simulink model "VehicleDynamics3D_traj"  (R2018a)
settings: Solver=ode15s  StartTime=0.0  StopTime=Stoptime  FixedStep=.001  MaxStep=maxStep  RelTol=relTol  AbsTol=absTol  EnableMultiTasking=on
PreLoadFcn:
  | VehicleDynamicsInitialization.m
model workspace: external: MATLAB File C:\Users\Puspita\Desktop\VehicleDynamics\sm_suspension_templates_params_ori.m (data not in the file)
values from neighbouring files (symbols this model uses):
  contactDamping = 1200    [VehicleDynamicsInitialization.m]    (also in traj1_results.mat)
  contactStiffness = 1E+6    (= 1000000)    [VehicleDynamicsInitialization.m]    (also in traj1_results.mat)
  dwb =     [modelworkspace.mat]    (also in sm_suspension_templates_params_ref.m = struct)
  Floor =     [traj1_results.mat]
  followerCameraX = 7.5    [VehicleDynamicsInitialization.m]    (also in traj1_results.mat)
  followerCameraZ = 3    [VehicleDynamicsInitialization.m]    (also in traj1_results.mat)
  frontCameraX = -1.75    [VehicleDynamicsInitialization.m]    (also in traj1_results.mat)
  frontCameraZ = 0.35    [VehicleDynamicsInitialization.m]    (also in traj1_results.mat)
  isoCameraAimX = (1/2)*wheelbase    (= 0.75)    [VehicleDynamicsInitialization.m]    (also in traj1_results.mat)
  isoCameraX = -3.1    [VehicleDynamicsInitialization.m]    (also in traj1_results.mat)
  isoCameraY = 3.5    [VehicleDynamicsInitialization.m]    (also in traj1_results.mat)
  isoCameraZ = 1.5    [VehicleDynamicsInitialization.m]    (also in traj1_results.mat)
  kineticFrictionCoeff = 0.88    [VehicleDynamicsInitialization.m]    (also in traj1_results.mat)
  limit = 105    [Run_Rear_Ident.m]    (also in test_traj.m = 50; traj1_results.mat = 50)
  Load = 200*scale    (= 200)    [VehicleDynamicsInitialization.m]    (also in traj1_results.mat)
  m = 200    [test_2.mat]    (also in test_traj.mat; test_traj2.mat; traj1_results.mat; traj_8.mat)
  maxSteeringDisplacement = 12    [VehicleDynamicsInitialization.m]    (also in traj1_results.mat = 10)
  minSteeringDisplacement = -12    [VehicleDynamicsInitialization.m]    (also in traj1_results.mat = -10)
  SetPaceSampleTime = 0.1    [VehicleDynamicsInitialization.m]    (also in traj1_results.mat)
  staticFrictionCoeff = 0.90    (= 0.9)    [VehicleDynamicsInitialization.m]    (also in traj1_results.mat)
  steeringInput = 0    [VehicleDynamicsInitialization.m]    (also in traj1_results.mat)
  vehicleSpeed_kph = 0    [VehicleDynamicsInitialization.m]    (also in traj1_results.mat)
  velocityThreshold = 1.5    [VehicleDynamicsInitialization.m]    (also in traj1_results.mat)
  wheel =     [modelworkspace.mat]    (also in sm_suspension_templates_params_ref.m = struct; traj1_results.mat)
  wheelbase = 1.5*scale    (= 1.5)    [VehicleDynamicsInitialization.m]    (also in traj1_results.mat)
undefined symbols (not defined in the file or in its folder): sigbuilder_block, X, Y, Z
libraries: sm_lib x237, nesl_utility x83, sm_suspension_templates_lib x34, Contact_Forces_Lib x16, simulink x12, fl_lib x1, aerolibanimutils x1
(part 5 of 10)

== system VehicleDynamics3D_traj/FrontSuspension/Chassis Assembly ==
  Back Frame : sm_suspension_templates_lib/Trapezoidal Frame  L1=dwb.chassis.frame.longlength  L2=dwb.chassis.frame.shortlength  H=dwb.chassis.frame.height  R=dwb.chassis.frame.cornerradius  T=dwb.chassis.frame.thickness  Tb=dwb.chassis.frame.barthickness  rho=dwb.chassis.frame.density  clr=dwb.chassis.frame.color
  DL Link : sm_suspension_templates_lib/Link 3  L=dwb.chassis.lowerlink.length  Ro=dwb.chassis.lowerlink.outerradius  Ri=dwb.chassis.lowerlink.innerradius  Lw=dwb.chassis.lowerlink.wishboneslotlength  Ld=dwb.chassis.lowerlink.wishboneseparation  Ow=dwb.chassis.lowerlink.wishboneoffset  Rr=dwb.chassis.lowerlink.chamferradius  rho=dwb.chassis.lowerlink.density  clr=dwb.chassis.lowerlink.color
  DR Link : sm_suspension_templates_lib/Link 3  L=dwb.chassis.lowerlink.length  Ro=dwb.chassis.lowerlink.outerradius  Ri=dwb.chassis.lowerlink.innerradius  Lw=dwb.chassis.lowerlink.wishboneslotlength  Ld=dwb.chassis.lowerlink.wishboneseparation  Ow=dwb.chassis.lowerlink.wishboneoffset  Rr=dwb.chassis.lowerlink.chamferradius  rho=dwb.chassis.lowerlink.density  clr=dwb.chassis.lowerlink.color
  Front Frame : Subsystem  mask(Trapeziodal Frame){L1=dwb.chassis.frame.longlength, L2=dwb.chassis.frame.shortlength, H=dwb.chassis.frame.height, R=dwb.chassis.frame.cornerradius, T=dwb.chassis.frame.thickness, Tb=dwb.chassis.frame.barthickness, rho=dwb.chassis.frame.density, clr=dwb.chassis.frame.color}
      mask prompts: L1 "Long side length of frame (cm):"; L2 "Short side length of frame (cm):"; H "Height of frame (cm):"; R "Radius of rounded corners (cm):"; T "Thickness of frame (cm):"; Tb "Thickness of frame bars (cm):"; rho "Density (kg/m^3):"; clr "Color ([r g b]):"
      mask help: This block models a trapeziodal frame that is part of the chassis on to which the suspension is mounted. The ports DR, DL, UR, UL correspond to the four corners of the frame. The port R corresponds to the central reference frame.
      mask init:
      | phi = atan2(H,(L1-L2)/2);
      | 
      | outer_xsec = [L2/2 -H/2; L1/2 H/2; -L1/2 H/2; -L2/2 -H/2];
      | 
      | inner_xsec = [ L2/2-Tb/tan((pi-phi)/2)    -(H/2-Tb);
      |                -L2/2+Tb/tan((pi-phi)/2)   -(H/2-Tb);
      |                -L1/2+Tb/tan(phi/2)          H/2-Tb;
      |                L1/2-Tb/tan(phi/2)           H/2-Tb];
      | 
      | % Frames are midway between the inner and outer 
      | % trapezium vertices           
      | frames = (outer_xsec+[inner_xsec(1,:); flipud(inner_xsec(2:end,:))])/2;
      | 
      | outer_xsec = simmechanics.demohelpers.round_corners(outer_xsec,[1 2 3 4],R,20);
      | inner_xsec = simmechanics.demohelpers.round_corners(inner_xsec,[1 2 3 4],R,20);       
      |           
      | frame_xsec = [outer_xsec; outer_xsec(1,:); ...
      |               inner_xsec; inner_xsec(1,:)];      
      |           
      | sec = frames(1,:);          
      | nec = frames(2,:);          
      | nwc = frames(3,:);          
      | swc = frames(4,:);
      mask DialogControl ParameterTabVar0 Prompt: Dimensions
      mask DialogControl ParameterTabVar01 Prompt: Material Properties
      mask Display:
      | image(imread(fullfile(matlabroot,...
      |     'toolbox','physmod','sm','smdemos',...
      |     'suspension_templates','images','sm_isuspension_frame.png')));
      | 
      | port_label('LConn',1,'UL');
      | port_label('LConn',2,'DL');
      | port_label('LConn',3,'DR');
      | port_label('LConn',4,'UR');
  Load : Subsystem
  NE Damp Joint : sm_lib/Joints/Revolute Joint  SenseConstraintForce=off  SenseConstraintForceX=off  SenseConstraintForceY=off  SenseConstraintForceZ=off  SenseConstraintTorque=off  SenseConstraintTorqueX=off  SenseConstraintTorqueY=off  SenseConstraintTorqueZ=off  SenseTotalForce=off  SenseTotalForceX=off  SenseTotalForceY=off  SenseTotalForceZ=off  SenseTotalTorque=off  SenseTotalTorqueX=off  SenseTotalTorqueY=off  SenseTotalTorqueZ=off  CompositeWrenchDir=FollowerOnBase  CompositeWrenchFrame=BaseFrame  EquilibriumPosition=0  EquilibriumPositionUnits=deg  SpringStiffness=0  SpringStiffnessUnits=N*m/deg  DampingCoefficient=0  DampingCoefficientUnits=N*m/(deg/s)  TorqueActuationMode=NoTorque  MotionActuationMode=ComputedMotion  SensePosition=off  SenseVelocity=off  SenseAcceleration=off  SenseTorqueForce=off  PositionTargetSpecify=off  PositionTargetPriority=High  PositionTargetValue=0  PositionTargetValueUnits=deg  VelocityTargetSpecify=off  VelocityTargetPriority=High  VelocityTargetValue=0  VelocityTargetValueUnits=deg/s
  NW Damp Joint : sm_lib/Joints/Revolute Joint  SenseConstraintForce=off  SenseConstraintForceX=off  SenseConstraintForceY=off  SenseConstraintForceZ=off  SenseConstraintTorque=off  SenseConstraintTorqueX=off  SenseConstraintTorqueY=off  SenseConstraintTorqueZ=off  SenseTotalForce=off  SenseTotalForceX=off  SenseTotalForceY=off  SenseTotalForceZ=off  SenseTotalTorque=off  SenseTotalTorqueX=off  SenseTotalTorqueY=off  SenseTotalTorqueZ=off  CompositeWrenchDir=FollowerOnBase  CompositeWrenchFrame=BaseFrame  EquilibriumPosition=0  EquilibriumPositionUnits=deg  SpringStiffness=0  SpringStiffnessUnits=N*m/deg  DampingCoefficient=0  DampingCoefficientUnits=N*m/(deg/s)  TorqueActuationMode=NoTorque  MotionActuationMode=ComputedMotion  SensePosition=off  SenseVelocity=off  SenseAcceleration=off  SenseTorqueForce=off  PositionTargetSpecify=off  PositionTargetPriority=High  PositionTargetValue=0  PositionTargetValueUnits=deg  VelocityTargetSpecify=off  VelocityTargetPriority=High  VelocityTargetValue=0  VelocityTargetValueUnits=deg/s
  Steering System : Subsystem
      mask Display:
      | image(imread(fullfile(matlabroot,...
      |     'toolbox','physmod','sm','smdemos',...
      |     'suspension_templates','images','sm_isuspension_steeringsys.png')))
      | 
      | port_label('LConn',1,'B');
      | port_label('RConn',1,'LT');
      | port_label('RConn',2,'RT');
  UL Link : sm_suspension_templates_lib/Link 1  L=dwb.chassis.upperlink.length  Ro=dwb.chassis.upperlink.outerradius  Ri=dwb.chassis.upperlink.innerradius  Lw=dwb.chassis.upperlink.wishboneslotlength  Ls=dwb.chassis.upperlink.springdamperslotlength  Ld=dwb.chassis.upperlink.wishboneseparation  Ow=dwb.chassis.upperlink.wishboneoffset  Rr=dwb.chassis.upperlink.chamferradius  rho=dwb.chassis.upperlink.density  clr=dwb.chassis.upperlink.color
  UR Link : sm_suspension_templates_lib/Link 1  L=dwb.chassis.upperlink.length  Ro=dwb.chassis.upperlink.outerradius  Ri=dwb.chassis.upperlink.innerradius  Lw=dwb.chassis.upperlink.wishboneslotlength  Ls=dwb.chassis.upperlink.springdamperslotlength  Ld=dwb.chassis.upperlink.wishboneseparation  Ow=dwb.chassis.upperlink.wishboneoffset  Rr=dwb.chassis.upperlink.chamferradius  rho=dwb.chassis.upperlink.density  clr=dwb.chassis.upperlink.color
  BC : PMIOPort  Side=Left
  ULA : PMIOPort  Port=2  Side=Left
  ULB : PMIOPort  Port=3  Side=Left
  ULC : PMIOPort  Port=4  Side=Left
  DLA : PMIOPort  Port=5  Side=Left
  DLB : PMIOPort  Port=6  Side=Left
  LT : PMIOPort  Port=7  Side=Left
  URA : PMIOPort  Port=8  Side=Right
  URB : PMIOPort  Port=9  Side=Right
  URC : PMIOPort  Port=10  Side=Right
  DRA : PMIOPort  Port=11  Side=Right
  DRB : PMIOPort  Port=12  Side=Right
  RT : PMIOPort  Port=13  Side=Right
  S : PMIOPort  Port=14  Side=Left
  connections:
  DR Link/LConn3 -- DRB/RConn1
  DR Link/LConn2 -- DRA/RConn1
  DLA/RConn1 -- DL Link/LConn2
  DLB/RConn1 -- DL Link/LConn3
  UR Link/LConn3 -- URB/RConn1
  UR Link/LConn2 -- URA/RConn1
  Front Frame/LConn2 -- DL Link/LConn1
  UR Link/LConn1 -- Front Frame/LConn4
  Back Frame/LConn2 -- DL Link/LConn4
  DR Link/LConn1 -- Front Frame/LConn3
  ULB/RConn1 -- UL Link/LConn3
  Back Frame/LConn3 -- DR Link/LConn4
  UR Link/LConn5 -- Back Frame/LConn4
  Back Frame/LConn1 -- UL Link/LConn5
  ULA/RConn1 -- UL Link/LConn2
  UL Link/LConn1 -- Front Frame/LConn1
  Back Frame/RConn1 -- Load/RConn1 -- Steering System/LConn1 -- BC/RConn1
  LT/RConn1 -- Steering System/RConn1
  Steering System/RConn2 -- RT/RConn1
  NW Damp Joint/LConn1 -- UL Link/LConn4
  NW Damp Joint/RConn1 -- ULC/RConn1
  NE Damp Joint/LConn1 -- UR Link/LConn4
  NE Damp Joint/RConn1 -- URC/RConn1
  S/RConn1 -- Steering System/LConn2

== system VehicleDynamics3D_traj/FrontSuspension/L Spr-Damp Assm ==
  Cyl Bracket : sm_suspension_templates_lib/Single Bracket  L=Lb  W=Wb  T=Tb  Rh=Rbh  rho=rho  clr=cclr
  Cyl Bracket XForm : sm_lib/Frames and Transforms/Rigid Transform  TranslationMethod=StandardAxis  TranslationStandardOffset=Lc/2  TranslationLengthUnit=cm  TranslationStandardAxis=-Z  TranslationCartesianOffset=[0 0 0]  TranslationROffset=0  TranslationROffsetUnits=m  TranslationZOffset=0  TranslationZOffsetUnits=m  TranslationThetaOffset=0  TranslationThetaOffsetUnits=deg  RotationMethod=AlignedAxes  RotationAngleUnits=deg  RotationStandardAxis=+Z  RotationAngle=0  RotationArbitraryAxis=[0 0 1]  FollAlignAxisA=+Z  BaseAlignAxisA=-Z  FollAlignAxisB=+X  BaseAlignAxisB=-X  RotationSequenceAxes=FollowerAxes  RotationSequence=XYX  RotationSequenceAngles=[0 0 0]  RotationSequenceAnglesUnits=deg  RotationMatrix=[1 0 0; 0 1 0; 0 0 1]
  Cyl-Piston Joint : sm_lib/Joints/Prismatic Joint  SenseConstraintForce=off  SenseConstraintForceX=off  SenseConstraintForceY=off  SenseConstraintForceZ=off  SenseConstraintTorque=off  SenseConstraintTorqueX=off  SenseConstraintTorqueY=off  SenseConstraintTorqueZ=off  SenseTotalForce=off  SenseTotalForceX=off  SenseTotalForceY=off  SenseTotalForceZ=off  SenseTotalTorque=off  SenseTotalTorqueX=off  SenseTotalTorqueY=off  SenseTotalTorqueZ=off  CompositeWrenchDir=FollowerOnBase  CompositeWrenchFrame=BaseFrame  EquilibriumPosition=Ls-(Lc-Lp)/2  EquilibriumPositionUnits=cm  SpringStiffness=Ks  SpringStiffnessUnits=N/m  DampingCoefficient=Kb  DampingCoefficientUnits=N/(m/s)  TorqueActuationMode=NoTorque  MotionActuationMode=ComputedMotion  SensePosition=on  SenseVelocity=off  SenseAcceleration=off  SenseTorqueForce=off  PositionTargetSpecify=off  PositionTargetPriority=Low  PositionTargetValue=Lp/2  PositionTargetValueUnits=cm  VelocityTargetSpecify=off  VelocityTargetPriority=High  VelocityTargetValue=0  VelocityTargetValueUnits=m/s
  Cylinder : sm_lib/Body Elements/Solid  InertiaType=CalculateFromGeometry  Mass=1  MassUnits=kg  CenterOfMass=[0 0 0]  CenterOfMassUnits=m  MomentsOfInertia=[1 1 1]  MomentsOfInertiaUnits=kg*m^2  ProductsOfInertia=[0 0 0]  ProductsOfInertiaUnits=kg*m^2  DensityBased=on  Density=rho  DensityUnits=kg/(m^3)  DoExposeReferenceFrame=on  SerializedFrames=<Frames/>  GraphicType=FromGeometry  MarkerShape=Sphere  MarkerSize=10  MarkerSizeUnits=m  GraphicVisPropType=SimpleVisualProperties  GraphicDiffuseColor=cclr  GraphicSpecularColor=[0.5 0.5 0.5 1.0]  GraphicAmbientColor=[0.15 0.15 0.15 1.0]  GraphicEmissiveColor=[0.0 0.0 0.0 1.0]  GraphicShininess=75  GraphicOpacity=0.75  GeometryShape=GeneralSolidOfRevolution  RectangleSize=[1 1]  RectangleSizeUnits=m  BrickDimensions=[1 1 1]  BrickDimensionUnits=m  CylinderRadius=1  CylinderRadiusUnits=m  CylinderLength=1  CylinderLengthUnits=m  SphereRadius=1  SphereRadiusUnits=m  EllipsoidRadii=[1 1 1]  EllipsoidRadiiUnits=m  ExtrusionCrossSection=[1 1; -1 1; -1 -1; 1 -1]  ExtrusionCrossSectionUnits=m  ExtrusionLength=1  ExtrusionLengthUnits=m  PolygonNumSides=3  PolygonOuterRadius=1  PolygonOuterRadiusUnits=m  ExtGeomFileType=STL  ExtGeomFileUnits=m  RevolutionCrossSection=cyl_xsec  RevolutionCrossSectionUnits=cm  RevolutionExtent=Full  RevolutionAngle=180  RevolutionAngleUnits=deg
  PS-Simulink Converter : nesl_utility/PS-Simulink Converter  PhysicalDomain=network_engine_domain  SubClassName=ps_output  LeftPortType=input  RightPortType=output  PseudoPeriodic=off  Frequencies=[]  Unit=cm  AffineConversion=off
  Pistion Bracket : sm_suspension_templates_lib/Single Bracket  L=Lb  W=Wb  T=Tb  Rh=Rbh  rho=rho  clr=pclr
  Piston : sm_lib/Body Elements/Solid  InertiaType=CalculateFromGeometry  Mass=1  MassUnits=kg  CenterOfMass=[0 0 0]  CenterOfMassUnits=m  MomentsOfInertia=[1 1 1]  MomentsOfInertiaUnits=kg*m^2  ProductsOfInertia=[0 0 0]  ProductsOfInertiaUnits=kg*m^2  DensityBased=on  Density=rho  DensityUnits=kg/(m^3)  DoExposeReferenceFrame=on  SerializedFrames=<Frames/>  GraphicType=FromGeometry  MarkerShape=Sphere  MarkerSize=10  MarkerSizeUnits=m  GraphicVisPropType=SimpleVisualProperties  GraphicDiffuseColor=pclr  GraphicSpecularColor=[0.5 0.5 0.5 1.0]  GraphicAmbientColor=[0.15 0.15 0.15 1.0]  GraphicEmissiveColor=[0.0 0.0 0.0 1.0]  GraphicShininess=75  GraphicOpacity=1  GeometryShape=GeneralSolidOfRevolution  RectangleSize=[1 1]  RectangleSizeUnits=m  BrickDimensions=[1 1 1]  BrickDimensionUnits=m  CylinderRadius=1  CylinderRadiusUnits=m  CylinderLength=1  CylinderLengthUnits=m  SphereRadius=1  SphereRadiusUnits=m  EllipsoidRadii=[1 1 1]  EllipsoidRadiiUnits=m  ExtrusionCrossSection=[1 1; -1 1; -1 -1; 1 -1]  ExtrusionCrossSectionUnits=m  ExtrusionLength=1  ExtrusionLengthUnits=m  PolygonNumSides=3  PolygonOuterRadius=1  PolygonOuterRadiusUnits=m  ExtGeomFileType=STL  ExtGeomFileUnits=m  RevolutionCrossSection=piston_xsec  RevolutionCrossSectionUnits=cm  RevolutionExtent=Full  RevolutionAngle=180  RevolutionAngleUnits=deg
  Piston Bracket XForm : sm_lib/Frames and Transforms/Rigid Transform  TranslationMethod=StandardAxis  TranslationStandardOffset=Lp/2  TranslationLengthUnit=cm  TranslationStandardAxis=+Z  TranslationCartesianOffset=[0 0 0]  TranslationROffset=0  TranslationROffsetUnits=m  TranslationZOffset=0  TranslationZOffsetUnits=m  TranslationThetaOffset=0  TranslationThetaOffsetUnits=deg  RotationMethod=None  RotationAngleUnits=deg  RotationStandardAxis=+Z  RotationAngle=0  RotationArbitraryAxis=[0 0 1]  FollAlignAxisA=+Z  BaseAlignAxisA=+Z  FollAlignAxisB=+X  BaseAlignAxisB=-X  RotationSequenceAxes=FollowerAxes  RotationSequence=XYX  RotationSequenceAngles=[0 0 0]  RotationSequenceAnglesUnits=deg  RotationMatrix=[1 0 0; 0 1 0; 0 0 1]
  Terminator : Terminator
  P : PMIOPort  Side=Right
  C : PMIOPort  Port=2  Side=Left
  wires:
  PS-Simulink Converter/1 -> Terminator/1  "FLSuspensionTravel_cm"
  connections:
  C/RConn1 -- Cyl Bracket/LConn1
  Pistion Bracket/LConn1 -- P/RConn1
  Pistion Bracket/RConn1 -- Piston Bracket XForm/RConn1
  Cyl Bracket/RConn1 -- Cyl Bracket XForm/RConn1
  Cyl-Piston Joint/RConn1 -- Piston/RConn1 -- Piston Bracket XForm/LConn1
  Cylinder/RConn1 -- Cyl-Piston Joint/LConn1 -- Cyl Bracket XForm/LConn1
  Cyl-Piston Joint/RConn2 -- PS-Simulink Converter/LConn1

== system VehicleDynamics3D_traj/FrontSuspension/L Suspension Assembly ==
  Knuckle : sm_suspension_templates_lib/Knuckle  H=dwb.knuckle.height  L=dwb.knuckle.length  T=dwb.knuckle.thickness  Wpr=dwb.knuckle.wheelattachprojwidth  Hpr=dwb.knuckle.wheelattachprojheight  Wc=dwb.knuckle.wishboneconnectorwidth  Rd=dwb.knuckle.driveshaftradius  Hd=dwb.knuckle.driveshaftheight  Rr=dwb.knuckle.chamferradius  Rt=dwb.knuckle.transitionradius  Rb=dwb.knuckle.ball.radius  Rp=dwb.knuckle.pin.radius  Hp=dwb.knuckle.pin.height  Ls=dwb.knuckle.steerarm.length  Ws=dwb.knuckle.steerarm.width  Ts=dwb.knuckle.steerarm.thickness  Hsf=dwb.knuckle.steerarm.forkheight  Lsf=dwb.knuckle.steerarm.forklength  Osf=dwb.knuckle.steerarm.forkoffset  Rsp=dwb.knuckle.pinradius  Rsr=dwb.knuckle.chamferradius  Rev=on  rho=dwb.knuckle.density  clr=dwb.knuckle.color
  Lower Knuckle Joint : sm_lib/Joints/Spherical Joint  SenseConstraintForce=off  SenseConstraintForceX=off  SenseConstraintForceY=off  SenseConstraintForceZ=off  SenseConstraintTorque=off  SenseConstraintTorqueX=off  SenseConstraintTorqueY=off  SenseConstraintTorqueZ=off  SenseTotalForce=off  SenseTotalForceX=off  SenseTotalForceY=off  SenseTotalForceZ=off  SenseTotalTorque=off  SenseTotalTorqueX=off  SenseTotalTorqueY=off  SenseTotalTorqueZ=off  CompositeWrenchDir=FollowerOnBase  CompositeWrenchFrame=BaseFrame  DefPosRotationMethod=None  DefPosRotationAngleUnits=deg  DefPosRotationStandardAxis=+Z  DefPosRotationAngle=0  DefPosRotationArbitraryAxis=[0 0 1]  DefPosFollAlignAxisA=+X  DefPosBaseAlignAxisA=+Y  DefPosFollAlignAxisB=+Y  DefPosBaseAlignAxisB=+Z  DefPosRotationSequenceAxes=FollowerAxes  DefPosRotationSequence=XYX  DefPosRotationSequenceAngles=[0 0 0]  DefPosRotationSequenceAnglesUnits=deg  DefPosRotationMatrix=[1 0 0; 0 1 0; 0 0 1]  EqPosRotationMethod=None  EqPosRotationAngleUnits=deg  EqPosRotationStandardAxis=+Z  EqPosRotationAngle=0  EqPosRotationArbitraryAxis=[0 0 1]  EqPosFollAlignAxisA=+X  EqPosBaseAlignAxisA=+Y  EqPosFollAlignAxisB=+Y  EqPosBaseAlignAxisB=+Z  EqPosRotationSequenceAxes=FollowerAxes  EqPosRotationSequence=XYX  EqPosRotationSequenceAngles=[0 0 0]  EqPosRotationSequenceAnglesUnits=deg  EqPosRotationMatrix=[1 0 0; 0 1 0; 0 0 1]  SpringStiffness=0  SpringStiffnessUnits=N*m/deg  DampingCoefficient=0  DampingCoefficientUnits=N*m/(deg/s)  ActuateTorqueX=off  ActuateTorqueY=off  ActuateTorqueZ=off  ActuateTorque=off  TorqueActuationMode=NoTorque  MotionActuationMode=ComputedMotion  ActuationFrame=BaseFrame  SensePosition=off  SenseVelocityX=off  SenseVelocityY=off  SenseVelocityZ=off  SenseVelocity=off  SenseAccelerationX=off  SenseAccelerationY=off  SenseAccelerationZ=off  SenseAcceleration=off  SenseTorqueX=off  SenseTorqueY=off  SenseTorqueZ=off  SenseTorqueForce=off  SensingFrame=BaseFrame  PositionTargetRotationMethod=None  PositionTargetRotationAngleUnits=deg  PositionTargetRotationStandardAxis=+Z  PositionTargetRotationAngle=0  PositionTargetRotationArbitraryAxis=[0 0 1]  PositionTargetFollAlignAxisA=+Y  PositionTargetBaseAlignAxisA=-Y  PositionTargetFollAlignAxisB=+Z  PositionTargetBaseAlignAxisB=-Z  PositionTargetRotationSequenceAxes=FollowerAxes  PositionTargetRotationSequence=XYX  PositionTargetRotationSequenceAngles=[0 0 0]  PositionTargetRotationSequenceAnglesUnits=deg  PositionTargetRotationMatrix=[1 0 0; 0 1 0; 0 0 1]  PositionTargetSpecify=off  PositionTargetPriority=Low  VelocityTargetValue=[0 0 0]  VelocityTargetValueUnits=deg/s  VelocityTargetSpecify=off  VelocityTargetPriority=High  VelocityTargetInFollowerFrame=on
  Lower Wishbone : sm_suspension_templates_lib/Lower Wishbone  L1=dwb.lwb.longlength  L2=dwb.lwb.shortlength  L3=dwb.lwb.wheellinklength  W3=dwb.lwb.wheellinkwidth  W=dwb.lwb.width  T=dwb.lwb.thickness  Rb=dwb.lwb.baseradius  Ob=dwb.lwb.basearcoffset  Rev=on  Lb=dwb.lwb.bracket.length  Rsh=dwb.lwb.bracket.radius  Rs=dwb.lwb.socket.radius  Hi=dwb.lwb.socket.height  Rh=dwb.lwb.socket.holeradius  Oh=dwb.lwb.socket.holeoffset  Odb=dwb.lwb.damperbracket.offset  Wdb=dwb.lwb.damperbracket.width  Ldb=dwb.lwb.damperbracket.length  Tdb=dwb.lwb.damperbracket.thickness  Sdb=dwb.lwb.damperbracket.spacing  Rhdb=dwb.lwb.damperbracket.holeradius  rho=dwb.lwb.density  clr=dwb.lwb.color
  SW Damp Joint : sm_lib/Joints/Revolute Joint  SenseConstraintForce=off  SenseConstraintForceX=off  SenseConstraintForceY=off  SenseConstraintForceZ=off  SenseConstraintTorque=off  SenseConstraintTorqueX=off  SenseConstraintTorqueY=off  SenseConstraintTorqueZ=off  SenseTotalForce=off  SenseTotalForceX=off  SenseTotalForceY=off  SenseTotalForceZ=off  SenseTotalTorque=off  SenseTotalTorqueX=off  SenseTotalTorqueY=off  SenseTotalTorqueZ=off  CompositeWrenchDir=FollowerOnBase  CompositeWrenchFrame=BaseFrame  EquilibriumPosition=0  EquilibriumPositionUnits=deg  SpringStiffness=0  SpringStiffnessUnits=N*m/deg  DampingCoefficient=0  DampingCoefficientUnits=N*m/(deg/s)  TorqueActuationMode=NoTorque  MotionActuationMode=ComputedMotion  SensePosition=off  SenseVelocity=off  SenseAcceleration=off  SenseTorqueForce=off  PositionTargetSpecify=off  PositionTargetPriority=Low  PositionTargetValue=-30  PositionTargetValueUnits=deg  VelocityTargetSpecify=off  VelocityTargetPriority=High  VelocityTargetValue=0  VelocityTargetValueUnits=deg/s
  Upper Knuckle Joint : sm_lib/Joints/Spherical Joint  SenseConstraintForce=off  SenseConstraintForceX=off  SenseConstraintForceY=off  SenseConstraintForceZ=off  SenseConstraintTorque=off  SenseConstraintTorqueX=off  SenseConstraintTorqueY=off  SenseConstraintTorqueZ=off  SenseTotalForce=off  SenseTotalForceX=off  SenseTotalForceY=off  SenseTotalForceZ=off  SenseTotalTorque=off  SenseTotalTorqueX=off  SenseTotalTorqueY=off  SenseTotalTorqueZ=off  CompositeWrenchDir=FollowerOnBase  CompositeWrenchFrame=BaseFrame  DefPosRotationMethod=None  DefPosRotationAngleUnits=deg  DefPosRotationStandardAxis=+Z  DefPosRotationAngle=0  DefPosRotationArbitraryAxis=[0 0 1]  DefPosFollAlignAxisA=+X  DefPosBaseAlignAxisA=+Y  DefPosFollAlignAxisB=+Y  DefPosBaseAlignAxisB=+Z  DefPosRotationSequenceAxes=FollowerAxes  DefPosRotationSequence=XYX  DefPosRotationSequenceAngles=[0 0 0]  DefPosRotationSequenceAnglesUnits=deg  DefPosRotationMatrix=[1 0 0; 0 1 0; 0 0 1]  EqPosRotationMethod=None  EqPosRotationAngleUnits=deg  EqPosRotationStandardAxis=+Z  EqPosRotationAngle=0  EqPosRotationArbitraryAxis=[0 0 1]  EqPosFollAlignAxisA=+X  EqPosBaseAlignAxisA=+Y  EqPosFollAlignAxisB=+Y  EqPosBaseAlignAxisB=+Z  EqPosRotationSequenceAxes=FollowerAxes  EqPosRotationSequence=XYX  EqPosRotationSequenceAngles=[0 0 0]  EqPosRotationSequenceAnglesUnits=deg  EqPosRotationMatrix=[1 0 0; 0 1 0; 0 0 1]  SpringStiffness=0  SpringStiffnessUnits=N*m/deg  DampingCoefficient=0  DampingCoefficientUnits=N*m/(deg/s)  ActuateTorqueX=off  ActuateTorqueY=off  ActuateTorqueZ=off  ActuateTorque=off  TorqueActuationMode=NoTorque  MotionActuationMode=ComputedMotion  ActuationFrame=BaseFrame  SensePosition=off  SenseVelocityX=off  SenseVelocityY=off  SenseVelocityZ=off  SenseVelocity=off  SenseAccelerationX=off  SenseAccelerationY=off  SenseAccelerationZ=off  SenseAcceleration=off  SenseTorqueX=off  SenseTorqueY=off  SenseTorqueZ=off  SenseTorqueForce=off  SensingFrame=BaseFrame  PositionTargetRotationMethod=StandardAxis  PositionTargetRotationAngleUnits=deg  PositionTargetRotationStandardAxis=+Z  PositionTargetRotationAngle=0  PositionTargetRotationArbitraryAxis=[0 0 1]  PositionTargetFollAlignAxisA=+X  PositionTargetBaseAlignAxisA=-X  PositionTargetFollAlignAxisB=+Z  PositionTargetBaseAlignAxisB=-Z  PositionTargetRotationSequenceAxes=FollowerAxes  PositionTargetRotationSequence=XYX  PositionTargetRotationSequenceAngles=[0 0 0]  PositionTargetRotationSequenceAnglesUnits=deg  PositionTargetRotationMatrix=[1 0 0; 0 1 0; 0 0 1]  PositionTargetSpecify=off  PositionTargetPriority=High  VelocityTargetValue=[0 0 0]  VelocityTargetValueUnits=deg/s  VelocityTargetSpecify=off  VelocityTargetPriority=High  VelocityTargetInFollowerFrame=on
  Upper Wishbone : sm_suspension_templates_lib/Wishbone  L1=dwb.uwb.longlength  L2=dwb.uwb.shortlength  L3=dwb.uwb.wheellinklength  W3=dwb.uwb.wheellinkwidth  W=dwb.uwb.width  T=dwb.uwb.thickness  Rb=dwb.uwb.baseradius  Ob=dwb.uwb.basearcoffset  Rev=on  Lb=dwb.uwb.bracket.length  Rsh=dwb.uwb.bracket.radius  Rs=dwb.uwb.socket.radius  Hi=dwb.uwb.socket.height  Rh=dwb.uwb.socket.ballradius  Oh=dwb.uwb.socket.offset  rho=dwb.uwb.density  clr=dwb.uwb.color
  UA : PMIOPort  Side=Right
  UB : PMIOPort  Port=2  Side=Right
  T : PMIOPort  Port=3  Side=Left
  DP : PMIOPort  Port=4  Side=Right
  DA : PMIOPort  Port=5  Side=Right
  DB : PMIOPort  Port=6  Side=Right
  S : PMIOPort  Port=7  Side=Right
  connections:
  Lower Wishbone/RConn1 -- Lower Knuckle Joint/LConn1
  Knuckle/LConn1 -- T/RConn1
  Lower Wishbone/LConn3 -- DB/RConn1
  Lower Wishbone/LConn2 -- DA/RConn1
  Upper Wishbone/LConn1 -- UA/RConn1
  UB/RConn1 -- Upper Wishbone/LConn2
  S/RConn1 -- Knuckle/LConn2
  Knuckle/RConn2 -- Lower Knuckle Joint/RConn1
  SW Damp Joint/LConn1 -- Lower Wishbone/LConn1
  SW Damp Joint/RConn1 -- DP/RConn1
  Upper Knuckle Joint/LConn1 -- Upper Wishbone/RConn1
  Upper Knuckle Joint/RConn1 -- Knuckle/RConn1

== system VehicleDynamics3D_traj/FrontSuspension/R Spr-Damp Assm ==
  Cyl Bracket : sm_suspension_templates_lib/Single Bracket  L=Lb  W=Wb  T=Tb  Rh=Rbh  rho=rho  clr=cclr
  Cyl Bracket XForm : sm_lib/Frames and Transforms/Rigid Transform  TranslationMethod=StandardAxis  TranslationStandardOffset=Lc/2  TranslationLengthUnit=cm  TranslationStandardAxis=-Z  TranslationCartesianOffset=[0 0 0]  TranslationROffset=0  TranslationROffsetUnits=m  TranslationZOffset=0  TranslationZOffsetUnits=m  TranslationThetaOffset=0  TranslationThetaOffsetUnits=deg  RotationMethod=AlignedAxes  RotationAngleUnits=deg  RotationStandardAxis=+Z  RotationAngle=0  RotationArbitraryAxis=[0 0 1]  FollAlignAxisA=+Z  BaseAlignAxisA=-Z  FollAlignAxisB=+X  BaseAlignAxisB=-X  RotationSequenceAxes=FollowerAxes  RotationSequence=XYX  RotationSequenceAngles=[0 0 0]  RotationSequenceAnglesUnits=deg  RotationMatrix=[1 0 0; 0 1 0; 0 0 1]
  Cyl-Piston Joint : sm_lib/Joints/Prismatic Joint  SenseConstraintForce=off  SenseConstraintForceX=off  SenseConstraintForceY=off  SenseConstraintForceZ=off  SenseConstraintTorque=off  SenseConstraintTorqueX=off  SenseConstraintTorqueY=off  SenseConstraintTorqueZ=off  SenseTotalForce=off  SenseTotalForceX=off  SenseTotalForceY=off  SenseTotalForceZ=off  SenseTotalTorque=off  SenseTotalTorqueX=off  SenseTotalTorqueY=off  SenseTotalTorqueZ=off  CompositeWrenchDir=FollowerOnBase  CompositeWrenchFrame=BaseFrame  EquilibriumPosition=Ls-(Lc-Lp)/2  EquilibriumPositionUnits=cm  SpringStiffness=Ks  SpringStiffnessUnits=N/m  DampingCoefficient=Kb  DampingCoefficientUnits=N/(m/s)  TorqueActuationMode=NoTorque  MotionActuationMode=ComputedMotion  SensePosition=on  SenseVelocity=off  SenseAcceleration=off  SenseTorqueForce=off  PositionTargetSpecify=off  PositionTargetPriority=Low  PositionTargetValue=Lp/2  PositionTargetValueUnits=cm  VelocityTargetSpecify=off  VelocityTargetPriority=High  VelocityTargetValue=0  VelocityTargetValueUnits=m/s
  Cylinder : sm_lib/Body Elements/Solid  InertiaType=CalculateFromGeometry  Mass=1  MassUnits=kg  CenterOfMass=[0 0 0]  CenterOfMassUnits=m  MomentsOfInertia=[1 1 1]  MomentsOfInertiaUnits=kg*m^2  ProductsOfInertia=[0 0 0]  ProductsOfInertiaUnits=kg*m^2  DensityBased=on  Density=rho  DensityUnits=kg/(m^3)  DoExposeReferenceFrame=on  SerializedFrames=<Frames/>  GraphicType=FromGeometry  MarkerShape=Sphere  MarkerSize=10  MarkerSizeUnits=m  GraphicVisPropType=SimpleVisualProperties  GraphicDiffuseColor=cclr  GraphicSpecularColor=[0.5 0.5 0.5 1.0]  GraphicAmbientColor=[0.15 0.15 0.15 1.0]  GraphicEmissiveColor=[0.0 0.0 0.0 1.0]  GraphicShininess=75  GraphicOpacity=0.75  GeometryShape=GeneralSolidOfRevolution  RectangleSize=[1 1]  RectangleSizeUnits=m  BrickDimensions=[1 1 1]  BrickDimensionUnits=m  CylinderRadius=1  CylinderRadiusUnits=m  CylinderLength=1  CylinderLengthUnits=m  SphereRadius=1  SphereRadiusUnits=m  EllipsoidRadii=[1 1 1]  EllipsoidRadiiUnits=m  ExtrusionCrossSection=[1 1; -1 1; -1 -1; 1 -1]  ExtrusionCrossSectionUnits=m  ExtrusionLength=1  ExtrusionLengthUnits=m  PolygonNumSides=3  PolygonOuterRadius=1  PolygonOuterRadiusUnits=m  ExtGeomFileType=STL  ExtGeomFileUnits=m  RevolutionCrossSection=cyl_xsec  RevolutionCrossSectionUnits=cm  RevolutionExtent=Full  RevolutionAngle=180  RevolutionAngleUnits=deg
  PS-Simulink Converter : nesl_utility/PS-Simulink Converter  PhysicalDomain=network_engine_domain  SubClassName=ps_output  LeftPortType=input  RightPortType=output  PseudoPeriodic=off  Frequencies=[]  Unit=cm  AffineConversion=off
  Pistion Bracket : sm_suspension_templates_lib/Single Bracket  L=Lb  W=Wb  T=Tb  Rh=Rbh  rho=rho  clr=pclr
  Piston : sm_lib/Body Elements/Solid  InertiaType=CalculateFromGeometry  Mass=1  MassUnits=kg  CenterOfMass=[0 0 0]  CenterOfMassUnits=m  MomentsOfInertia=[1 1 1]  MomentsOfInertiaUnits=kg*m^2  ProductsOfInertia=[0 0 0]  ProductsOfInertiaUnits=kg*m^2  DensityBased=on  Density=rho  DensityUnits=kg/(m^3)  DoExposeReferenceFrame=on  SerializedFrames=<Frames/>  GraphicType=FromGeometry  MarkerShape=Sphere  MarkerSize=10  MarkerSizeUnits=m  GraphicVisPropType=SimpleVisualProperties  GraphicDiffuseColor=pclr  GraphicSpecularColor=[0.5 0.5 0.5 1.0]  GraphicAmbientColor=[0.15 0.15 0.15 1.0]  GraphicEmissiveColor=[0.0 0.0 0.0 1.0]  GraphicShininess=75  GraphicOpacity=1  GeometryShape=GeneralSolidOfRevolution  RectangleSize=[1 1]  RectangleSizeUnits=m  BrickDimensions=[1 1 1]  BrickDimensionUnits=m  CylinderRadius=1  CylinderRadiusUnits=m  CylinderLength=1  CylinderLengthUnits=m  SphereRadius=1  SphereRadiusUnits=m  EllipsoidRadii=[1 1 1]  EllipsoidRadiiUnits=m  ExtrusionCrossSection=[1 1; -1 1; -1 -1; 1 -1]  ExtrusionCrossSectionUnits=m  ExtrusionLength=1  ExtrusionLengthUnits=m  PolygonNumSides=3  PolygonOuterRadius=1  PolygonOuterRadiusUnits=m  ExtGeomFileType=STL  ExtGeomFileUnits=m  RevolutionCrossSection=piston_xsec  RevolutionCrossSectionUnits=cm  RevolutionExtent=Full  RevolutionAngle=180  RevolutionAngleUnits=deg
  Piston Bracket XForm : sm_lib/Frames and Transforms/Rigid Transform  TranslationMethod=StandardAxis  TranslationStandardOffset=Lp/2  TranslationLengthUnit=cm  TranslationStandardAxis=+Z  TranslationCartesianOffset=[0 0 0]  TranslationROffset=0  TranslationROffsetUnits=m  TranslationZOffset=0  TranslationZOffsetUnits=m  TranslationThetaOffset=0  TranslationThetaOffsetUnits=deg  RotationMethod=None  RotationAngleUnits=deg  RotationStandardAxis=+Z  RotationAngle=0  RotationArbitraryAxis=[0 0 1]  FollAlignAxisA=+Z  BaseAlignAxisA=+Z  FollAlignAxisB=+X  BaseAlignAxisB=-X  RotationSequenceAxes=FollowerAxes  RotationSequence=XYX  RotationSequenceAngles=[0 0 0]  RotationSequenceAnglesUnits=deg  RotationMatrix=[1 0 0; 0 1 0; 0 0 1]
  Terminator : Terminator
  P : PMIOPort  Side=Right
  C : PMIOPort  Port=2  Side=Left
  wires:
  PS-Simulink Converter/1 -> Terminator/1  "FRSuspensionTravel_cm"
  connections:
  C/RConn1 -- Cyl Bracket/LConn1
  Pistion Bracket/LConn1 -- P/RConn1
  Pistion Bracket/RConn1 -- Piston Bracket XForm/RConn1
  Cyl Bracket/RConn1 -- Cyl Bracket XForm/RConn1
  Cyl-Piston Joint/RConn1 -- Piston/RConn1 -- Piston Bracket XForm/LConn1
  Cylinder/RConn1 -- Cyl-Piston Joint/LConn1 -- Cyl Bracket XForm/LConn1
  Cyl-Piston Joint/RConn2 -- PS-Simulink Converter/LConn1

== system VehicleDynamics3D_traj/FrontSuspension/R Suspension Assembly ==
  Knuckle : sm_suspension_templates_lib/Knuckle  H=dwb.knuckle.height  L=dwb.knuckle.length  T=dwb.knuckle.thickness  Wpr=dwb.knuckle.wheelattachprojwidth  Hpr=dwb.knuckle.wheelattachprojheight  Wc=dwb.knuckle.wishboneconnectorwidth  Rd=dwb.knuckle.driveshaftradius  Hd=dwb.knuckle.driveshaftheight  Rr=dwb.knuckle.chamferradius  Rt=dwb.knuckle.transitionradius  Rb=dwb.knuckle.ball.radius  Rp=dwb.knuckle.pin.radius  Hp=dwb.knuckle.pin.height  Ls=dwb.knuckle.steerarm.length  Ws=dwb.knuckle.steerarm.width  Ts=dwb.knuckle.steerarm.thickness  Hsf=dwb.knuckle.steerarm.forkheight  Lsf=dwb.knuckle.steerarm.forklength  Osf=dwb.knuckle.steerarm.forkoffset  Rsp=dwb.knuckle.pinradius  Rsr=dwb.knuckle.chamferradius  Rev=off  rho=dwb.knuckle.density  clr=dwb.knuckle.color
  Lower Knuckle Joint : sm_lib/Joints/Spherical Joint  SenseConstraintForce=off  SenseConstraintForceX=off  SenseConstraintForceY=off  SenseConstraintForceZ=off  SenseConstraintTorque=off  SenseConstraintTorqueX=off  SenseConstraintTorqueY=off  SenseConstraintTorqueZ=off  SenseTotalForce=off  SenseTotalForceX=off  SenseTotalForceY=off  SenseTotalForceZ=off  SenseTotalTorque=off  SenseTotalTorqueX=off  SenseTotalTorqueY=off  SenseTotalTorqueZ=off  CompositeWrenchDir=FollowerOnBase  CompositeWrenchFrame=BaseFrame  DefPosRotationMethod=None  DefPosRotationAngleUnits=deg  DefPosRotationStandardAxis=+Z  DefPosRotationAngle=0  DefPosRotationArbitraryAxis=[0 0 1]  DefPosFollAlignAxisA=+X  DefPosBaseAlignAxisA=+Y  DefPosFollAlignAxisB=+Y  DefPosBaseAlignAxisB=+Z  DefPosRotationSequenceAxes=FollowerAxes  DefPosRotationSequence=XYX  DefPosRotationSequenceAngles=[0 0 0]  DefPosRotationSequenceAnglesUnits=deg  DefPosRotationMatrix=[1 0 0; 0 1 0; 0 0 1]  EqPosRotationMethod=None  EqPosRotationAngleUnits=deg  EqPosRotationStandardAxis=+Z  EqPosRotationAngle=0  EqPosRotationArbitraryAxis=[0 0 1]  EqPosFollAlignAxisA=+X  EqPosBaseAlignAxisA=+Y  EqPosFollAlignAxisB=+Y  EqPosBaseAlignAxisB=+Z  EqPosRotationSequenceAxes=FollowerAxes  EqPosRotationSequence=XYX  EqPosRotationSequenceAngles=[0 0 0]  EqPosRotationSequenceAnglesUnits=deg  EqPosRotationMatrix=[1 0 0; 0 1 0; 0 0 1]  SpringStiffness=0  SpringStiffnessUnits=N*m/deg  DampingCoefficient=0  DampingCoefficientUnits=N*m/(deg/s)  ActuateTorqueX=off  ActuateTorqueY=off  ActuateTorqueZ=off  ActuateTorque=off  TorqueActuationMode=NoTorque  MotionActuationMode=ComputedMotion  ActuationFrame=BaseFrame  SensePosition=off  SenseVelocityX=off  SenseVelocityY=off  SenseVelocityZ=off  SenseVelocity=off  SenseAccelerationX=off  SenseAccelerationY=off  SenseAccelerationZ=off  SenseAcceleration=off  SenseTorqueX=off  SenseTorqueY=off  SenseTorqueZ=off  SenseTorqueForce=off  SensingFrame=BaseFrame  PositionTargetRotationMethod=None  PositionTargetRotationAngleUnits=deg  PositionTargetRotationStandardAxis=+Z  PositionTargetRotationAngle=0  PositionTargetRotationArbitraryAxis=[0 0 1]  PositionTargetFollAlignAxisA=+X  PositionTargetBaseAlignAxisA=-X  PositionTargetFollAlignAxisB=+Y  PositionTargetBaseAlignAxisB=-Y  PositionTargetRotationSequenceAxes=FollowerAxes  PositionTargetRotationSequence=XYX  PositionTargetRotationSequenceAngles=[0 0 0]  PositionTargetRotationSequenceAnglesUnits=deg  PositionTargetRotationMatrix=[1 0 0; 0 1 0; 0 0 1]  PositionTargetSpecify=off  PositionTargetPriority=Low  VelocityTargetValue=[0 0 0]  VelocityTargetValueUnits=deg/s  VelocityTargetSpecify=off  VelocityTargetPriority=High  VelocityTargetInFollowerFrame=on
  Lower Wishbone : sm_suspension_templates_lib/Lower Wishbone  L1=dwb.lwb.longlength  L2=dwb.lwb.shortlength  L3=dwb.lwb.wheellinklength  W3=dwb.lwb.wheellinkwidth  W=dwb.lwb.width  T=dwb.lwb.thickness  Rb=dwb.lwb.baseradius  Ob=dwb.lwb.basearcoffset  Rev=off  Lb=dwb.lwb.bracket.length  Rsh=dwb.lwb.bracket.radius  Rs=dwb.lwb.socket.radius  Hi=dwb.lwb.socket.height  Rh=dwb.lwb.socket.holeradius  Oh=dwb.lwb.socket.holeoffset  Odb=dwb.lwb.damperbracket.offset  Wdb=dwb.lwb.damperbracket.width  Ldb=dwb.lwb.damperbracket.length  Tdb=dwb.lwb.damperbracket.thickness  Sdb=dwb.lwb.damperbracket.spacing  Rhdb=dwb.lwb.damperbracket.holeradius  rho=dwb.lwb.density  clr=dwb.lwb.color
  SE Damp Joint : sm_lib/Joints/Revolute Joint  SenseConstraintForce=off  SenseConstraintForceX=off  SenseConstraintForceY=off  SenseConstraintForceZ=off  SenseConstraintTorque=off  SenseConstraintTorqueX=off  SenseConstraintTorqueY=off  SenseConstraintTorqueZ=off  SenseTotalForce=off  SenseTotalForceX=off  SenseTotalForceY=off  SenseTotalForceZ=off  SenseTotalTorque=off  SenseTotalTorqueX=off  SenseTotalTorqueY=off  SenseTotalTorqueZ=off  CompositeWrenchDir=FollowerOnBase  CompositeWrenchFrame=BaseFrame  EquilibriumPosition=0  EquilibriumPositionUnits=deg  SpringStiffness=0  SpringStiffnessUnits=N*m/deg  DampingCoefficient=0  DampingCoefficientUnits=N*m/(deg/s)  TorqueActuationMode=NoTorque  MotionActuationMode=ComputedMotion  SensePosition=off  SenseVelocity=off  SenseAcceleration=off  SenseTorqueForce=off  PositionTargetSpecify=off  PositionTargetPriority=Low  PositionTargetValue=150  PositionTargetValueUnits=deg  VelocityTargetSpecify=off  VelocityTargetPriority=High  VelocityTargetValue=0  VelocityTargetValueUnits=deg/s
  Upper Knuckle Joint : sm_lib/Joints/Spherical Joint  SenseConstraintForce=off  SenseConstraintForceX=off  SenseConstraintForceY=off  SenseConstraintForceZ=off  SenseConstraintTorque=off  SenseConstraintTorqueX=off  SenseConstraintTorqueY=off  SenseConstraintTorqueZ=off  SenseTotalForce=off  SenseTotalForceX=off  SenseTotalForceY=off  SenseTotalForceZ=off  SenseTotalTorque=off  SenseTotalTorqueX=off  SenseTotalTorqueY=off  SenseTotalTorqueZ=off  CompositeWrenchDir=FollowerOnBase  CompositeWrenchFrame=BaseFrame  DefPosRotationMethod=None  DefPosRotationAngleUnits=deg  DefPosRotationStandardAxis=+Z  DefPosRotationAngle=0  DefPosRotationArbitraryAxis=[0 0 1]  DefPosFollAlignAxisA=+X  DefPosBaseAlignAxisA=+Y  DefPosFollAlignAxisB=+Y  DefPosBaseAlignAxisB=+Z  DefPosRotationSequenceAxes=FollowerAxes  DefPosRotationSequence=XYX  DefPosRotationSequenceAngles=[0 0 0]  DefPosRotationSequenceAnglesUnits=deg  DefPosRotationMatrix=[1 0 0; 0 1 0; 0 0 1]  EqPosRotationMethod=None  EqPosRotationAngleUnits=deg  EqPosRotationStandardAxis=+Z  EqPosRotationAngle=0  EqPosRotationArbitraryAxis=[0 0 1]  EqPosFollAlignAxisA=+X  EqPosBaseAlignAxisA=+Y  EqPosFollAlignAxisB=+Y  EqPosBaseAlignAxisB=+Z  EqPosRotationSequenceAxes=FollowerAxes  EqPosRotationSequence=XYX  EqPosRotationSequenceAngles=[0 0 0]  EqPosRotationSequenceAnglesUnits=deg  EqPosRotationMatrix=[1 0 0; 0 1 0; 0 0 1]  SpringStiffness=0  SpringStiffnessUnits=N*m/deg  DampingCoefficient=0  DampingCoefficientUnits=N*m/(deg/s)  ActuateTorqueX=off  ActuateTorqueY=off  ActuateTorqueZ=off  ActuateTorque=off  TorqueActuationMode=NoTorque  MotionActuationMode=ComputedMotion  ActuationFrame=BaseFrame  SensePosition=off  SenseVelocityX=off  SenseVelocityY=off  SenseVelocityZ=off  SenseVelocity=off  SenseAccelerationX=off  SenseAccelerationY=off  SenseAccelerationZ=off  SenseAcceleration=off  SenseTorqueX=off  SenseTorqueY=off  SenseTorqueZ=off  SenseTorqueForce=off  SensingFrame=BaseFrame  PositionTargetRotationMethod=StandardAxis  PositionTargetRotationAngleUnits=deg  PositionTargetRotationStandardAxis=+Z  PositionTargetRotationAngle=0  PositionTargetRotationArbitraryAxis=[0 0 1]  PositionTargetFollAlignAxisA=+X  PositionTargetBaseAlignAxisA=-X  PositionTargetFollAlignAxisB=+Y  PositionTargetBaseAlignAxisB=-Y  PositionTargetRotationSequenceAxes=FollowerAxes  PositionTargetRotationSequence=XYX  PositionTargetRotationSequenceAngles=[0 0 0]  PositionTargetRotationSequenceAnglesUnits=deg  PositionTargetRotationMatrix=[1 0 0; 0 1 0; 0 0 1]  PositionTargetSpecify=off  PositionTargetPriority=High  VelocityTargetValue=[0 0 0]  VelocityTargetValueUnits=deg/s  VelocityTargetSpecify=off  VelocityTargetPriority=High  VelocityTargetInFollowerFrame=on
  Upper Wishbone : sm_suspension_templates_lib/Wishbone  L1=dwb.uwb.longlength  L2=dwb.uwb.shortlength  L3=dwb.uwb.wheellinklength  W3=dwb.uwb.wheellinkwidth  W=dwb.uwb.width  T=dwb.uwb.thickness  Rb=dwb.uwb.baseradius  Ob=dwb.uwb.basearcoffset  Rev=off  Lb=dwb.uwb.bracket.length  Rsh=dwb.uwb.bracket.radius  Rs=dwb.uwb.socket.radius  Hi=dwb.uwb.socket.height  Rh=dwb.uwb.socket.ballradius  Oh=dwb.uwb.socket.offset  rho=dwb.uwb.density  clr=dwb.uwb.color
  UA : PMIOPort  Side=Left
  UB : PMIOPort  Port=2  Side=Left
  T : PMIOPort  Port=3  Side=Right
  DP : PMIOPort  Port=4  Side=Left
  DA : PMIOPort  Port=5  Side=Left
  DB : PMIOPort  Port=6  Side=Left
  S : PMIOPort  Port=7  Side=Left
  connections:
  Lower Wishbone/RConn1 -- Lower Knuckle Joint/LConn1
  Lower Wishbone/LConn3 -- DB/RConn1
  Lower Wishbone/LConn2 -- DA/RConn1
  UA/RConn1 -- Upper Wishbone/LConn1
  Lower Knuckle Joint/RConn1 -- Knuckle/RConn2
  UB/RConn1 -- Upper Wishbone/LConn2
  S/RConn1 -- Knuckle/LConn2
  DP/RConn1 -- SE Damp Joint/LConn1
  SE Damp Joint/RConn1 -- Lower Wishbone/LConn1
  T/RConn1 -- Knuckle/LConn1
  Upper Wishbone/RConn1 -- Upper Knuckle Joint/LConn1
  Upper Knuckle Joint/RConn1 -- Knuckle/RConn1

== system VehicleDynamics3D_traj/Inputs/SpeedProcessing ==
  V : Inport
  Integrator : Integrator
  OtherWheel : Gain  Gain=-1
  Simulink-PS Converter : nesl_utility/Simulink-PS Converter  PhysicalDomain=network_engine_domain  SubClassName=ps_input  LeftPortType=input  RightPortType=output  PseudoPeriodic=off  Frequencies=[]  NoiseDistribution=none  NoiseParameters=[]  Unit=rad  AffineConversion=off  FilteringAndDerivatives=filter  SimscapeFilterOrder=2  InputFilterTimeConstant=wheelFilterTimeConst  UdotUserProvided=0
  Simulink-PS Converter1 : nesl_utility/Simulink-PS Converter  PhysicalDomain=network_engine_domain  SubClassName=ps_input  LeftPortType=input  RightPortType=output  PseudoPeriodic=off  Frequencies=[]  NoiseDistribution=none  NoiseParameters=[]  Unit=rad  AffineConversion=off  FilteringAndDerivatives=filter  SimscapeFilterOrder=2  InputFilterTimeConstant=wheelFilterTimeConst  UdotUserProvided=0
  To Workspace2 : ToWorkspace  VariableName=velocity_input  SampleTime=-1
  mps2mph : Subsystem
  wheelRadius_m : Gain  Gain=1/(wheel.tire.outerradius*.01)
      settings: AttributesFormatString=%<Gain>
  L : PMIOPort  Side=Right
  R : PMIOPort  Port=2  Side=Right
  wires:
  Integrator/1 -> To Workspace2/1, OtherWheel/1, Simulink-PS Converter/1
  OtherWheel/1 -> Simulink-PS Converter1/1
  mps2mph/1(V[mps]) -> wheelRadius_m/1
  wheelRadius_m/1 -> Integrator/1
  V/1 -> mps2mph/1(V[kph])
  connections:
  Simulink-PS Converter1/RConn1 -- R/RConn1
  Simulink-PS Converter/RConn1 -- L/RConn1

== system VehicleDynamics3D_traj/Inputs/SteeringProcessing ==
  S : Inport
  Saturation : Saturate  UpperLimit=maxSteeringDisplacement  LowerLimit=minSteeringDisplacement
  Simulink-PS Converter : nesl_utility/Simulink-PS Converter  PhysicalDomain=network_engine_domain  SubClassName=ps_input  LeftPortType=input  RightPortType=output  PseudoPeriodic=off  Frequencies=[]  NoiseDistribution=none  NoiseParameters=[]  Unit=cm  AffineConversion=off  FilteringAndDerivatives=filter  SimscapeFilterOrder=2  InputFilterTimeConstant=steeringFilterTimeConst  UdotUserProvided=2
  To Workspace1 : ToWorkspace  VariableName=steering_input  SampleTime=-1
  PsS : PMIOPort  Side=Right
  wires:
  S/1 -> Saturation/1
  Saturation/1 -> To Workspace1/1, Simulink-PS Converter/1
  connections:
  Simulink-PS Converter/RConn1 -- PsS/RConn1

== system VehicleDynamics3D_traj/Inputs/User Input ==
  Burnout : Subsystem  VariantControl=BurnoutVariant
  "DashboardInput " : Subsystem  VariantControl=DashboardVariant
  LeftTurn90 : Subsystem  VariantControl=LeftTurnVariant
  RightTurn90 : Subsystem  VariantControl=RightTurnVariant
  Skidpad : Subsystem  VariantControl=SkidpadVariant
  Slalom : Subsystem  VariantControl=(default)
  SteepSteer : Subsystem  VariantControl=SteepSteerVariant
  Steering : Outport
  Speed : Outport  Port=2
